simulink model "A1_MPC_AttitudeDynamics"  (R2017b)
settings: Solver=VariableStepAuto  StartTime=0.0  StopTime=20  FixedStep=1  MaxStep=0.1  RelTol=1e-6  EnableMultiTasking=on
PostLoadFcn:
  | AttitudeDynamicsData;
StopFcn:
  | attitudePlot = animateAttitude(rotmOut, 0.016);
  | attitudePlot.plotInit;
  | responsePlot(responseData, rotmOut, omegaRsOut, mechEnergyOut, mechPowerOut, torqueOut);
  | %fprintf(2, 'max torque [mNm]: %5.2f', sqrt(max(torqueOut.Data(:,1).^2+torqueOut.Data(:,2).^2+torqueOut.Data(:,3).^2))*1000)
values from neighbouring files (symbols this model uses):
  J_sat = [2.5 2.5 2.5]    [AttitudeDynamicsData.m]
  PID_MPC = struct(      'P', 1.3,          'I', 0.0002,     'D', 3.02           )    [AttitudeDynamicsData.m]
  T_disturb = ones(1,3) * 0.1E-3    [AttitudeDynamicsData.m]
undefined symbols (not defined in the file or in its folder): DiscIntNeverNeededParam
libraries: SatelliteLibrary x15, mpclib x1, simulink x1
(part 2 of 2)

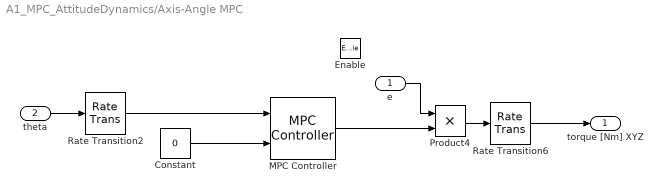
== system A1_MPC_AttitudeDynamics/Axis-Angle MPC ==
  e : Inport
  theta : Inport  Port=2
  Enable : EnablePort  StatesWhenEnabling=reset
  Constant : Constant  Value=0
  MPC Controller : mpclib/MPC Controller  SCDEnableBlockLinearizationSpecification=on  mpcobj=mpc1  is_multiple=0  enable_value=0  return_u0=off  ref_from_ws=off  ref_signal_name=[]  ref_preview=off  md_from_ws=off  md_signal_name=[]  md_preview=off  from_project=off  project_file=MPCtask.mat  md_inport=off  mv_inport=off  cost_outport=off  return_sequence=off  return_qpstatus=off  return_state=off  state_inport=off  lims_inport=off  cc_inport=off  ywt_inport=off  is_designfromscratch=0  uwt_inport=off  duwt_inport=off  rhoeps_inport=off  uref_inport=off  n_ts=1  n_p=20  n_mv=1  n_md=0  n_ud=0  n_mo=1  n_uo=0  BlockDataType=double  SampleTimeInherited=off  switch_inport=off
  Product4 : Product
  Rate Transition2 : RateTransition  OutPortSampleTime=tMPC
  Rate Transition6 : RateTransition  OutPortSampleTimeOpt=Inherit  OutPortSampleTime=1
  torque [Nm] XYZ : Outport
  wires:
  e/1 -> Product4/1
  Product4/1 -> Rate Transition6/1
  MPC Controller/1 -> Product4/2
  Rate Transition2/1 -> MPC Controller/1
  Constant/1 -> MPC Controller/2
  theta/1 -> Rate Transition2/1
  Rate Transition6/1 -> torque [Nm] XYZ/1

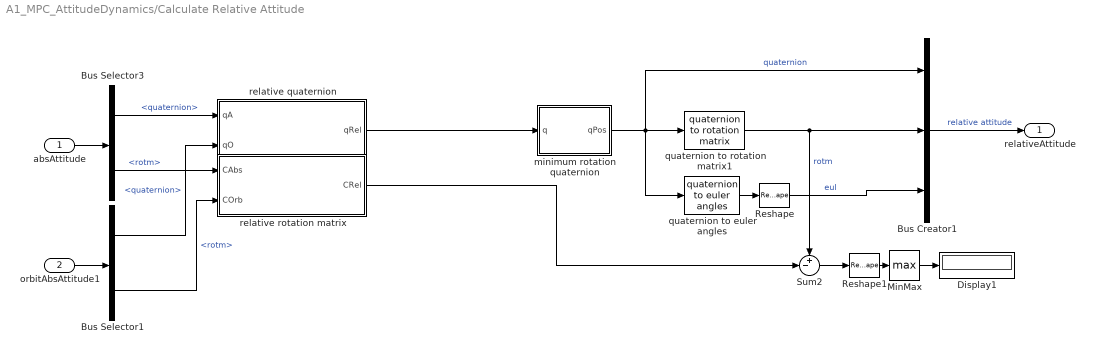
== system A1_MPC_AttitudeDynamics/Calculate Relative Attitude ==
  absAttitude : Inport
  orbitAbsAttitude1 : Inport  Port=2
  Bus Creator1 : BusCreator  Inputs=3
  Bus Selector1 : BusSelector  OutputSignals=quaternion,rotm
  Bus Selector3 : BusSelector  OutputSignals=quaternion,rotm
  Display1 : Display
  MinMax : MinMax  Function=max  ZeroCross=off
  Reshape : Reshape
  Reshape1 : Reshape
  Sum2 : Sum  Inputs=+-|
  minimum rotation quaternion : MATLAB Function  TreatAsAtomicUnit=on
  quaternion to euler angles : SatelliteLibrary/quaternion to euler angles
  quaternion to rotation matrix1 : SatelliteLibrary/quaternion to rotation matrix
  relative quaternion : MATLAB Function  TreatAsAtomicUnit=on
  relative rotation matrix : MATLAB Function  TreatAsAtomicUnit=on
  relativeAttitude : Outport
  wires:
  Bus Selector1/1 -> relative quaternion/2(qO)  "<quaternion>"
  Bus Selector3/2 -> relative rotation matrix/1(CAbs)  "<rotm>"
  Reshape1/1 -> MinMax/1
  MinMax/1 -> Display1/1
  relative rotation matrix/1(CRel) -> Sum2/2
  quaternion to rotation matrix1/1 -> Sum2/1, Bus Creator1/2  "rotm"
  Bus Creator1/1 -> relativeAttitude/1  "relative attitude"
  minimum rotation quaternion/1(qPos) -> Bus Creator1/1, quaternion to euler angles/1, quaternion to rotation matrix1/1  "quaternion"
  quaternion to euler angles/1 -> Reshape/1
  Bus Selector3/1 -> relative quaternion/1(qA)  "<quaternion>"
  Sum2/1 -> Reshape1/1
  relative quaternion/1(qRel) -> minimum rotation quaternion/1(q)
  Bus Selector1/2 -> relative rotation matrix/2(COrb)  "<rotm>"
  absAttitude/1 -> Bus Selector3/1
  orbitAbsAttitude1/1 -> Bus Selector1/1
  Reshape/1 -> Bus Creator1/3  "eul"

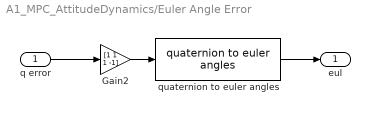
== system A1_MPC_AttitudeDynamics/Euler Angle Error ==
  q error : Inport
  Gain2 : Gain  Gain=[1 1 1 -1]
  quaternion to euler angles : SatelliteLibrary/quaternion to euler angles
  eul : Outport
  wires:
  quaternion to euler angles/1 -> eul/1
  q error/1 -> Gain2/1
  Gain2/1 -> quaternion to euler angles/1

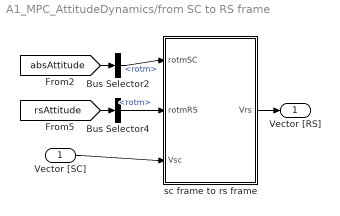
== system A1_MPC_AttitudeDynamics/from SC to RS frame ==
  Vector [SC] : Inport
  Bus Selector2 : BusSelector  OutputSignals=rotm
  Bus Selector4 : BusSelector  OutputSignals=rotm
  sc frame to rs frame : MATLAB Function  TreatAsAtomicUnit=on
  Vector [RS] : Outport
  wires:
  Vector [SC]/1 -> sc frame to rs frame/3(Vsc)
  sc frame to rs frame/1(Vrs) -> Vector [RS]/1
  [rsAttitude] -> Bus Selector4/1
  Bus Selector4/1 -> sc frame to rs frame/2(rotmRS)  "<rotm>"
  [absAttitude] -> Bus Selector2/1
  Bus Selector2/1 -> sc frame to rs frame/1(rotmSC)  "<rotm>"

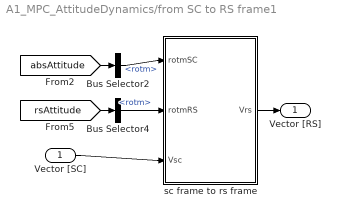
== system A1_MPC_AttitudeDynamics/from SC to RS frame1 ==
  Vector [SC] : Inport
  Bus Selector2 : BusSelector  OutputSignals=rotm
  Bus Selector4 : BusSelector  OutputSignals=rotm
  sc frame to rs frame : MATLAB Function  TreatAsAtomicUnit=on
  Vector [RS] : Outport
  wires:
  Vector [SC]/1 -> sc frame to rs frame/3(Vsc)
  sc frame to rs frame/1(Vrs) -> Vector [RS]/1
  [rsAttitude] -> Bus Selector4/1
  Bus Selector4/1 -> sc frame to rs frame/2(rotmRS)  "<rotm>"
  [absAttitude] -> Bus Selector2/1
  Bus Selector2/1 -> sc frame to rs frame/1(rotmSC)  "<rotm>"

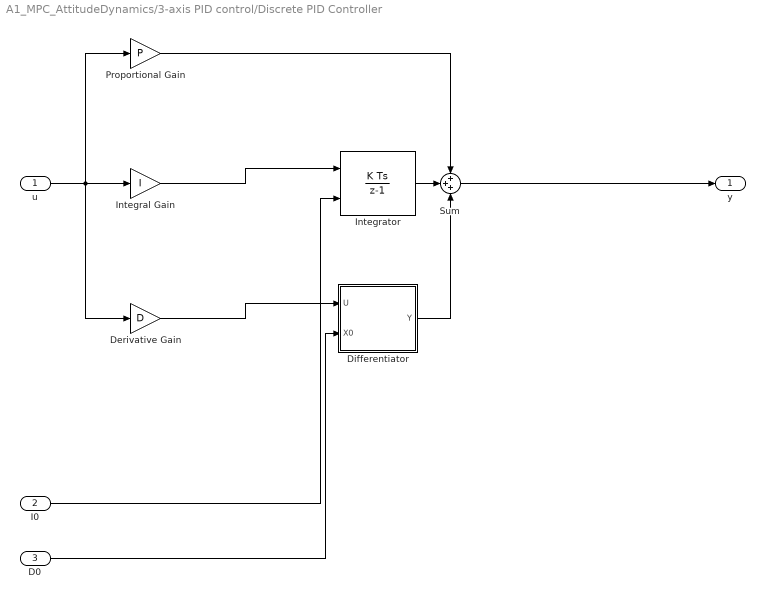
== system A1_MPC_AttitudeDynamics/3-axis PID control/Discrete PID Controller ==
  u : Inport  SampleTime=SampleTime
  I0 : Inport  Port=2  SampleTime=SampleTime
  D0 : Inport  Port=3  SampleTime=SampleTime
  Derivative Gain : Gain  DisableCoverage=on  Gain=D  ParamMin=DParamMin  ParamMax=DParamMax  OutMin=DOutMin  OutMax=DOutMax  SampleTime=SampleTime
  Differentiator : Subsystem
      mask Display: text(0.5, 0.5, '(z-1)', 'horizontalAlignment', 'center', 'verticalAlignment', 'bottom');text(0.5, 0.5, 'Ts z', 'horizontalAlignment', 'center', 'verticalAlignment', 'top');plot([0.3 0.7],[0.5 0.5]);port_label('input', 2, '\rmx_0', 'texmode', 'on');
  Integral Gain : Gain  DisableCoverage=on  Gain=I  ParamMin=IParamMin  ParamMax=IParamMax  OutMin=IOutMin  OutMax=IOutMax  SampleTime=SampleTime
  Integrator : DiscreteIntegrator  InitialConditionSource=external  InitialCondition=InitialConditionForIntegrator  InitialConditionSetting=State (most efficient)  SampleTime=SampleTime  OutMin=IntegratorOutMin  OutMax=IntegratorOutMax  ICPrevOutput=DiscIntNeverNeededParam  ICPrevScaledInput=DiscIntNeverNeededParam
  Proportional Gain : Gain  Gain=P  ParamMin=PParamMin  ParamMax=PParamMax  OutMin=POutMin  OutMax=POutMax  SampleTime=SampleTime
  Sum : Sum  Inputs=+++  OutMin=SumOutMin  OutMax=SumOutMax  SampleTime=SampleTime
  y : Outport  SampleTime=SampleTime  InitialOutput=0
  wires:
  u/1 -> Integral Gain/1, Derivative Gain/1, Proportional Gain/1
  Integral Gain/1 -> Integrator/1
  Integrator/1 -> Sum/2
  Derivative Gain/1 -> Differentiator/1(U)
  Differentiator/1(Y) -> Sum/3
  Proportional Gain/1 -> Sum/1
  Sum/1 -> y/1
  I0/1 -> Integrator/2
  D0/1 -> Differentiator/2(X0)

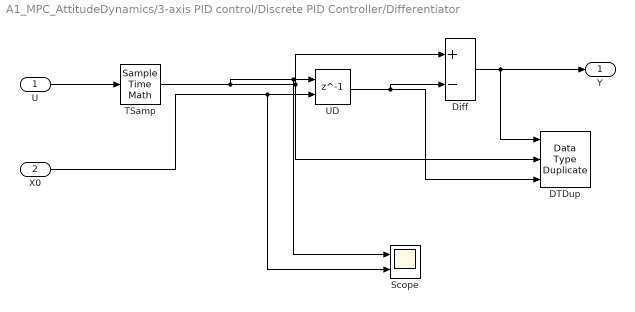
== system A1_MPC_AttitudeDynamics/3-axis PID control/Discrete PID Controller/Differentiator ==
  U : Inport  SampleTime=SampleTime
  X0 : Inport  Port=2
  DTDup : DataTypeDuplicate  NumInputPorts=3
  Diff : Sum  Inputs=+-  OutMin=DifferentiatorOutMin  OutMax=DifferentiatorOutMax  OutDataTypeStr=Inherit: Inherit via back propagation  InputSameDT=on
  Scope : Scope  NumInputPorts=2
  TSamp : SampleTimeMath  TsampMathOp=/  TsampMathImp=Offline Scaling Adjustment
  UD : Delay  DelayLength=1  InitialConditionSource=Input port  InitialCondition=DifferentiatorICPrevScaledInput  InputProcessing=Inherited
      settings: InputPortMap=u0,p4
  Y : Outport  OutMin=DifferentiatorOutMin  OutMax=DifferentiatorOutMax  SampleTime=SampleTime
  wires:
  U/1 -> TSamp/1
  TSamp/1 -> Diff/1, DTDup/2, Scope/1, UD/1
  UD/1 -> Diff/2, DTDup/3
  Diff/1 -> Y/1, DTDup/1
  X0/1 -> Scope/2, UD/2

== matlab function A1_MPC_AttitudeDynamics/Calculate Relative Attitude/minimum rotation quaternion ==
  data: q input; qPos output
function qPos = minRotation(q)
    % converts quaternion to form of smalest angle (last element always <0, 1] )
    if q(4) < 0
        qPos = -q;
    else
        qPos = q;
    end
end

== matlab function A1_MPC_AttitudeDynamics/from SC to RS frame/sc frame to rs frame ==
  data: rotmSC input; Vrs output; rotmRS input; Vsc input
function ...
    Vrs               ...
  = sc2rs(            ...
    rotmSC,         ...
    rotmRS,         ...
    Vsc             ...
    )
    % transform vector in spacecraft (SC) frame into vector in
    % reactionsphere (RS) frame.
    Vrs = rotmRS' * rotmSC * Vsc;

end

== matlab function A1_MPC_AttitudeDynamics/Calculate Relative Attitude/relative rotation matrix ==
  data: CAbs input; COrb input; CRel output
function CRel = rotmatRelative(...
    CAbs, ... absolute rotation matrix orientation (in inertial reference frame)
    COrb  ... orbital frame rotation matrix orientation
    )

CRel = COrb' * CAbs;
end

== matlab function A1_MPC_AttitudeDynamics/Axis Angle Error/minimum rotation quaternion ==
  data: q input; qPos output
function qPos = minRotation(q)
    % converts quaternion to form of smalest angle (last element always <0, 1] )
    if q(4) < 0
        qPos = -q;
    else
        qPos = q;
    end
end

== matlab function A1_MPC_AttitudeDynamics/Calculate Relative Attitude/relative quaternion ==
  data: qA input; qO input; qRel output
function qRel = quatRelative(...
    qA, ... absolute quaternion orientation (in inertial reference frame)
    qO  ... orbital frame quaternion orientation
    )
% Calculate the error quaternion
% q_... are standard quaternions with the vector part at the start

qOinv = [-qO(1:3); qO(4)];
qAmatrix = [ qA(4)  qA(3) -qA(2)  qA(1);...
            -qA(3)  qA(4)  qA(1)  qA(2);...
             qA(2) -qA(1)  qA(4)  qA(3);...
            -qA(1) -qA(2) -qA(3)  qA(4)];
qRel = qAmatrix * qOinv;
end

== matlab function A1_MPC_AttitudeDynamics/from SC to RS frame1/sc frame to rs frame ==
  data: rotmSC input; Vrs output; rotmRS input; Vsc input
function ...
    Vrs               ...
  = sc2rs(            ...
    rotmSC,         ...
    rotmRS,         ...
    Vsc             ...
    )
    % transform vector in spacecraft (SC) frame into vector in
    % reactionsphere (RS) frame.
    Vrs = rotmRS' * rotmSC * Vsc;

end
